simulink model "MDriverRegenRequested"  (R2024b)
settings: configuration reference "STM32H7_Config" (kept outside this file)
undefined symbols (not defined in the file): IRegen2C, IRegen6C, MNominal, MTotalMinAllowed, NKe, tMaxRegen, tTorqueControlTask
libraries: simulink x3
settings Model: DataDictionary=Master_Dictionary.sldd  EnableAccessToBaseWorkspace=off  Creator=torni  LastModifiedBy=William
settings ConfigSetRef: SourceName=STM32H7_Config

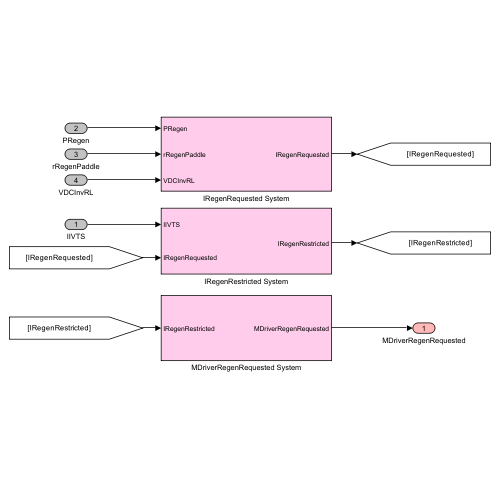
[thumbnail: Simulink's stored preview of the top-level diagram]
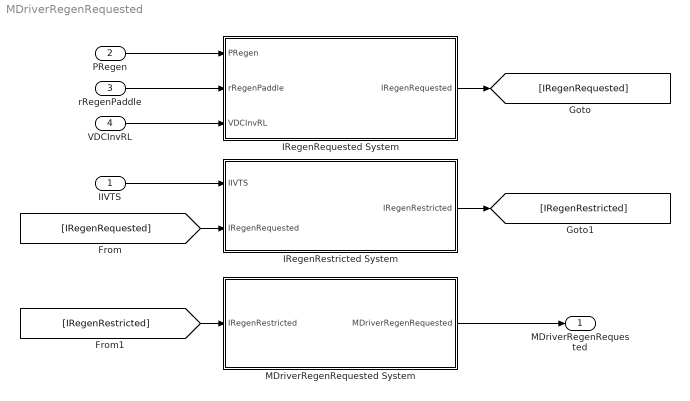
== system MDriverRegenRequested ==
  IIVTS : Inport  OutDataTypeStr=double
  PRegen : Inport  Port=2  OutDataTypeStr=double
  rRegenPaddle : Inport  Port=3  OutDataTypeStr=double
  VDCInvRL : Inport  Port=4  OutDataTypeStr=double
  IRegenRequested System : Subsystem
  IRegenRestricted System : Subsystem
  "MDriverRegenRequested System " : Subsystem
  MDriverRegenRequested : Outport  OutDataTypeStr=double  VectorParamsAs1DForOutWhenUnconnected=off
  wires:
  PRegen/1 -> IRegenRequested System/1(PRegen)
  rRegenPaddle/1 -> IRegenRequested System/2(rRegenPaddle)
  IIVTS/1 -> IRegenRestricted System/1(IIVTS)
  IRegenRequested System/1(IRegenRequested) -> [IRegenRequested]
  [IRegenRequested] -> IRegenRestricted System/2(IRegenRequested)
  IRegenRestricted System/1(IRegenRestricted) -> [IRegenRestricted]
  [IRegenRestricted] -> "MDriverRegenRequested System "/1(IRegenRestricted)
  "MDriverRegenRequested System "/1(MDriverRegenRequested) -> MDriverRegenRequested/1
  VDCInvRL/1 -> IRegenRequested System/3(VDCInvRL)

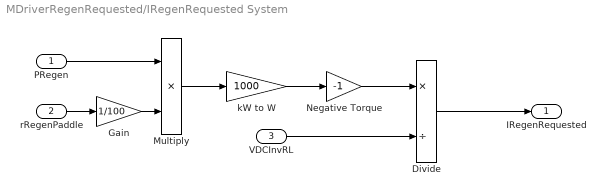
== system MDriverRegenRequested/IRegenRequested System ==
  PRegen : Inport  OutDataTypeStr=double
  rRegenPaddle : Inport  Port=2  OutDataTypeStr=double
  VDCInvRL : Inport  Port=3  OutDataTypeStr=double
  Divide : Product  Inputs=*/
  Gain : Gain  Gain=1/100
  Multiply : Product
  Negative Torque : Gain  Gain=-1
  kW to W : Gain  Gain=1000
  IRegenRequested : Outport  OutDataTypeStr=double  VectorParamsAs1DForOutWhenUnconnected=off
  wires:
  Negative Torque/1 -> Divide/1
  PRegen/1 -> Multiply/1
  kW to W/1 -> Negative Torque/1
  Multiply/1 -> kW to W/1
  Divide/1 -> IRegenRequested/1
  Gain/1 -> Multiply/2
  rRegenPaddle/1 -> Gain/1
  VDCInvRL/1 -> Divide/2

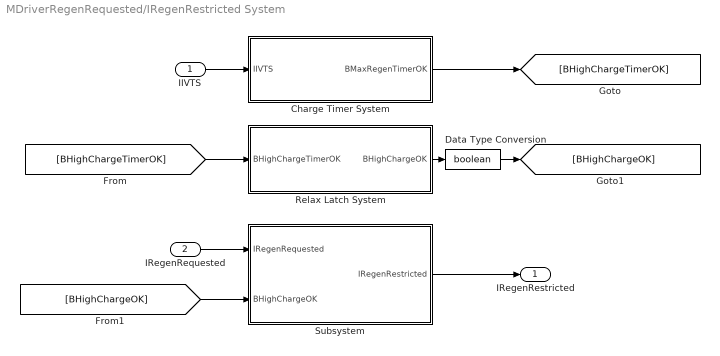
== system MDriverRegenRequested/IRegenRestricted System ==
  IIVTS : Inport  OutDataTypeStr=double
  IRegenRequested : Inport  Port=2  OutDataTypeStr=double
  Charge Timer System : Subsystem
  Data Type Conversion : DataTypeConversion  OutDataTypeStr=boolean  SaturateOnIntegerOverflow=off  RndMeth=Floor
  Relax Latch System : Stateflow chart  TreatAsAtomicUnit=on
  Subsystem : Subsystem
  IRegenRestricted : Outport  OutDataTypeStr=double  VectorParamsAs1DForOutWhenUnconnected=off
  wires:
  IIVTS/1 -> Charge Timer System/1(IIVTS)
  Charge Timer System/1(BMaxRegenTimerOK) -> [BHighChargeTimerOK]
  [BHighChargeTimerOK] -> Relax Latch System/1(BHighChargeTimerOK)
  IRegenRequested/1 -> Subsystem/1(IRegenRequested)
  [BHighChargeOK] -> Subsystem/2(BHighChargeOK)
  Subsystem/1(IRegenRestricted) -> IRegenRestricted/1
  Relax Latch System/1(BHighChargeOK) -> Data Type Conversion/1
  Data Type Conversion/1 -> [BHighChargeOK]

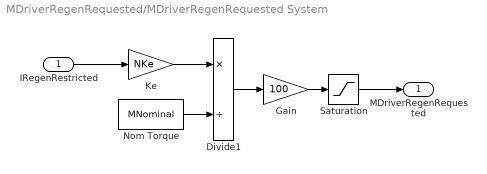
== system MDriverRegenRequested/MDriverRegenRequested System  ==
  IRegenRestricted : Inport
  Divide1 : Product  Inputs=*/
  Gain : Gain  Gain=100
  Ke : Gain  Gain=NKe
  Nom Torque : Constant  Value=MNominal
  Saturation : Saturate  UpperLimit=0  LowerLimit=MTotalMinAllowed
  MDriverRegenRequested : Outport  VectorParamsAs1DForOutWhenUnconnected=off
  wires:
  Nom Torque/1 -> Divide1/2
  Divide1/1 -> Gain/1
  IRegenRestricted/1 -> Ke/1
  Ke/1 -> Divide1/1
  Gain/1 -> Saturation/1
  Saturation/1 -> MDriverRegenRequested/1

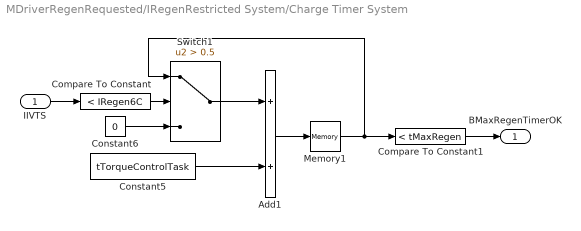
== system MDriverRegenRequested/IRegenRestricted System/Charge Timer System ==
  IIVTS : Inport  OutDataTypeStr=double
  Add1 : Sum
  Compare To Constant : simulink/Logic and Bit Operations/Compare To Constant  relop=<  const=IRegen6C  OutDataTypeStr=boolean
  Compare To Constant1 : simulink/Logic and Bit Operations/Compare To Constant  relop=<  const=tMaxRegen  OutDataTypeStr=boolean
  Constant5 : Constant  Value=tTorqueControlTask
  Constant6 : Constant  Value=0
  Memory1 : Memory  InheritSampleTime=on
  Switch1 : Switch  Criteria=u2 > Threshold  Threshold=0.5  SaturateOnIntegerOverflow=off  InputSameDT=off
  BMaxRegenTimerOK : Outport  OutDataTypeStr=boolean  VectorParamsAs1DForOutWhenUnconnected=off
  wires:
  Compare To Constant1/1 -> BMaxRegenTimerOK/1
  Memory1/1 -> Compare To Constant1/1, Switch1/1
  Switch1/1 -> Add1/1
  Add1/1 -> Memory1/1
  Compare To Constant/1 -> Switch1/2
  Constant5/1 -> Add1/2
  Constant6/1 -> Switch1/3
  IIVTS/1 -> Compare To Constant/1

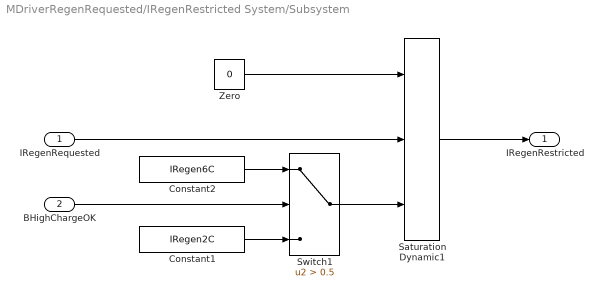
== system MDriverRegenRequested/IRegenRestricted System/Subsystem ==
  IRegenRequested : Inport  OutDataTypeStr=double
  BHighChargeOK : Inport  Port=2  OutDataTypeStr=boolean
  Constant1 : Constant  Value=IRegen2C
  Constant2 : Constant  Value=IRegen6C
  Saturation Dynamic1 : simulink/Discontinuities/Saturation Dynamic  OutMin=[]  OutMax=[]  OutDataTypeStr=Inherit: Same as second input  OutDataType=fixdt(1, 16)  OutScaling=2^-10  DoSatur=off
  Switch1 : Switch  Criteria=u2 > Threshold  Threshold=0.5  SaturateOnIntegerOverflow=off  InputSameDT=off
  Zero : Constant  Value=0  SampleTime=-1
  IRegenRestricted : Outport  OutDataTypeStr=double  VectorParamsAs1DForOutWhenUnconnected=off
  wires:
  Saturation Dynamic1/1 -> IRegenRestricted/1
  Switch1/1 -> Saturation Dynamic1/3
  IRegenRequested/1 -> Saturation Dynamic1/2
  Constant1/1 -> Switch1/3
  Constant2/1 -> Switch1/1
  Zero/1 -> Saturation Dynamic1/1
  BHighChargeOK/1 -> Switch1/2

== stateflow chart MDriverRegenRequested/IRegenRestricted System/Relax Latch System ==
  state Reset
    BHighChargeOK = 0;
  state Entrance
    entry:
    BHighChargeOK = 1;
  Entrance -> Reset : [BHighChargeTimerOK<0.5]
  (default) -> Entrance
  Reset -> Entrance : after(8000,tick)
  data: BHighChargeTimerOK input boolean; BHighChargeOK output double
